simulink model "BiorlWalkingBipedRobot copy"  (R2023b)
settings: Solver=ode23t  StartTime=0.0  StopTime=inf  RelTol=1e-2  EnableMultiTasking=on
undefined symbols (not defined in the file or in its folder): foot_z, height_plane, init_angs_R, init_height, joint_stiffness, lower_leg_length, max_torque, plane_x, plane_y, Tf, Ts, upper_leg_length, wx0, wy0, X, Y, Z
libraries: sm_lib x38, nesl_utility x25, walkingRobotUtils x4, simulink x2, rllib x1
(part 1 of 2)
settings Model: Creator=The MathWorks, Inc.  LastModifiedBy=amelianelson
settings SolverCC: ZeroCrossAlgorithm=Adaptive  AlgebraicLoopSolver=TrustRegion
settings DataIOCC: SaveOutput=off  SignalLogging=off  DSMLogging=off  SaveTime=off  OutputTimes=0:0.01:10
settings OptimizationCC: LifeSpan=inf
settings DebuggingCC: MaxConsecutiveZCsMsg=warning  IgnoredZcDiagnostic=none  UnconnectedInputMsg=warning  UnconnectedOutputMsg=warning  UnconnectedLineMsg=warning  AllowSymbolicDim=off  SFUnexpectedBacktrackingDiag=warning  SFNoUnconditionalDefaultTransitionDiag=warning  SFExecutionAtInitializationDiag=none  UnitsInconsistencyMsg=none  ArithmeticOperatorsInVariantConditions=warning
settings ModelReferenceCC: EnableRefExpFcnMdlSchedulingChecks=on
settings SFSimCC: SimUseLocalCustomCode=off  CustomCodeUndefinedFunction=UseInterfaceOnly
settings RTWCC: RTWUseLocalCustomCode=off
settings CodeAppCC: StateflowObjectComments=on
settings GRTTargetCC: TargetLangStandard=C89/C90 (ANSI)
settings ConfigComp: CovMetricSettings=dw  CovSaveCumulativeToWorkspaceVar=on  CovSaveSingleToWorkspaceVar=on  CovExternalEMLEnable=off  CovSFcnEnable=off
settings SimscapeCC: SimscapeNormalizeSystem=off  SimscapeLogOpenViewer=on  SimscapeLogLimitData=off  SimscapeLogDataHistory=10000
settings ConfigurationSet: Description=SimMechanics 2G
settings DiagnosticsConfigSet: SimMechanicsRigidlyBoundBlock=none
settings ExplorerConfigSet: InternalSimMechanicsExplorerSettings="<ExplorerConfiguration><canonicalview>default</canonicalview><AnimationSetting><BasePlaybackSpeed>1.0</BasePlaybackSpeed><PlaybackSpeedFactor>1.0</PlaybackSpeedFactor></AnimationSetting><TilePanel><TileInfo><Tiles Columns=\"1\" Count=\"1\" Rows=\"1\"><Column Weight=\"1\"/><Row Weight=\"1\"/><Tile Height=\"1\" Width=\"1\" X=\"0\" Y=\"0\"/></Tiles></TileInfo><SceneInfo><SceneViewer><BGColor><R>0.60000002384185791</R><G>0.60000002384185791</G><B>0.60000002384185791</B></BGColor><Camera><DoPerspective>off</DoPerspective><Position><X>7.18002534815406079</X><Y>-8.21011991112170847</Y><Z>8.33180938462712462</Z></Position><Center><X>1.10741005252516134</X><Y>-0.176829942633513204</Y><Z>0.646464709811595872</Z></Center><Up><X>-0.335329266167064488</X><Y>0.506481739462631531</Y><Z>0.79437430147428989</Z></Up><ViewLimDist>1</ViewLimDist><YLim>0.739205014828661411</YLim><XLim>1.12849377732657596</XLim></Camera></SceneViewer></SceneInfo></TilePanel><MechEditorPanel><Cameras/><GfxPanelCameraMap/><VideoCreator><PlaybackSpeedRatio>1.0</PlaybackSpeedRatio><FrameRate>30</FrameRate><VideoFormat>Motion JPEG AVI</VideoFormat><FrameSize>auto</FrameSize></VideoCreator></MechEditorPanel></ExplorerConfiguration>"

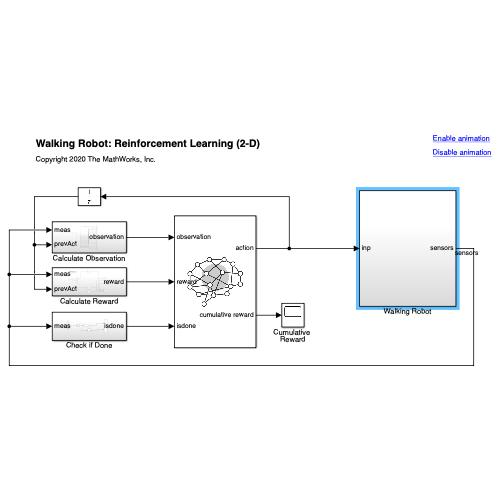
[thumbnail: Simulink's stored preview of the top-level diagram]
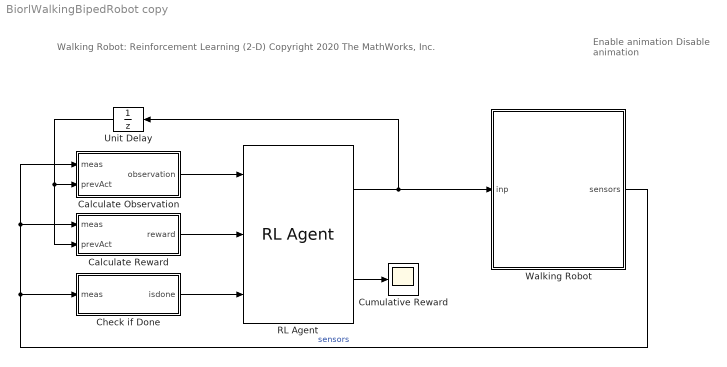
== system BiorlWalkingBipedRobot copy ==
  note: Enable animation
      |
      | Disable animation
  note: Walking Robot: Reinforcement Learning (2-D)
      |
      | Copyright 2020 The MathWorks, Inc.
  Calculate Observation : Subsystem
  Calculate Reward : Subsystem
  Check if Done : Subsystem
  Cumulative Reward : Scope
  RL Agent : rllib/RL Agent  Agent=agent  ExternalActionAsInput=off  ProvideLastAction=off  ProvideCumRwd=on  TreatAsDirectFeedthrough=on  UseStrictObservationDataTypes=off
  Unit Delay : UnitDelay  SampleTime=-1  HasFrameUpgradeWarning=on
  Walking Robot : Subsystem
  wires:
  Walking Robot/1(sensors) -> Calculate Reward/1(meas), Calculate Observation/1(meas), Check if Done/1(meas)  "sensors"
  Calculate Reward/1(reward) -> RL Agent/2
  Calculate Observation/1(observation) -> RL Agent/1
  Check if Done/1(isdone) -> RL Agent/3
  RL Agent/2 -> Cumulative Reward/1
  Unit Delay/1 -> Calculate Reward/2(prevAct), Calculate Observation/2(prevAct)
  RL Agent/1 -> Walking Robot/1(inp), Unit Delay/1

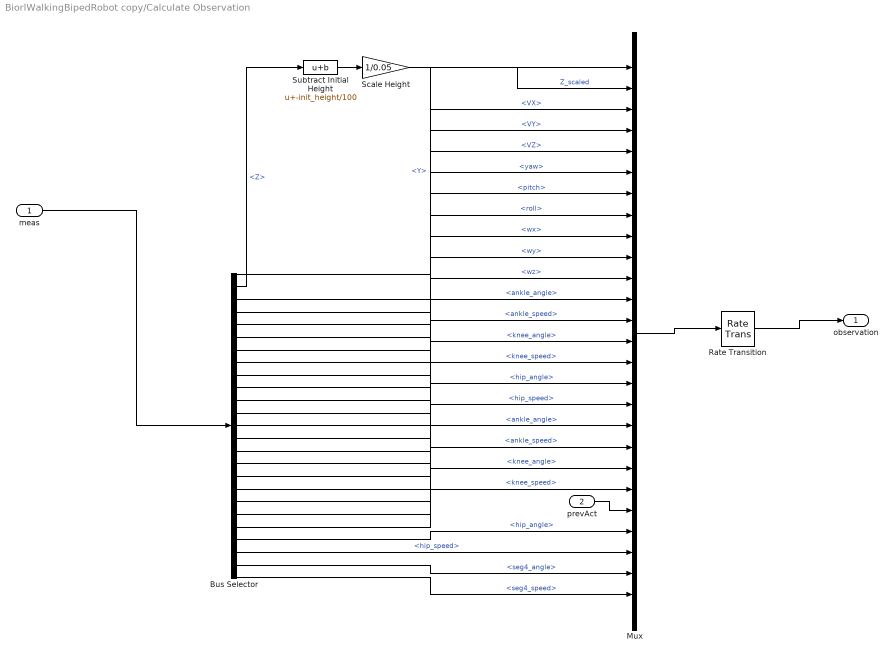
== system BiorlWalkingBipedRobot copy/Calculate Observation ==
  meas : Inport
  prevAct : Inport  Port=2
  Bus Selector : BusSelector  OutputSignals=Y,Z,VX,VY,VZ,yaw,pitch,roll,wx,wy,wz,measR.ankle_angle,measR.ankle_speed,measR.knee_angle,measR.knee_speed,measR.hip_angle,measR.hip_speed,measR.ankle_angle,measR.ankle_speed,measR.knee_angle,measR.knee_speed,measR.hip_angle,measR.hip_speed,measR.seg4_angle,measR.seg4_speed
  Mux : Mux  Inputs=26
  Rate Transition : RateTransition
  Scale Height : Gain  Gain=1/0.05
  Subtract Initial Height : Bias  Bias=-init_height/100  SaturateOnIntegerOverflow=off
  observation : Outport  VectorParamsAs1DForOutWhenUnconnected=off
  wires:
  meas/1 -> Bus Selector/1
  Mux/1 -> Rate Transition/1
  Rate Transition/1 -> observation/1
  prevAct/1 -> Mux/22
  Bus Selector/2 -> Subtract Initial Height/1  "<Z>"
  Subtract Initial Height/1 -> Scale Height/1
  Scale Height/1 -> Mux/2  "Z_scaled"
  Bus Selector/1 -> Mux/1  "<Y>"
  Bus Selector/4 -> Mux/4  "<VY>"
  Bus Selector/5 -> Mux/5  "<VZ>"
  Bus Selector/3 -> Mux/3  "<VX>"
  Bus Selector/6 -> Mux/6  "<yaw>"
  Bus Selector/7 -> Mux/7  "<pitch>"
  Bus Selector/8 -> Mux/8  "<roll>"
  Bus Selector/9 -> Mux/9  "<wx>"
  Bus Selector/10 -> Mux/10  "<wy>"
  Bus Selector/11 -> Mux/11  "<wz>"
  Bus Selector/12 -> Mux/12  "<ankle_angle>"
  Bus Selector/13 -> Mux/13  "<ankle_speed>"
  Bus Selector/14 -> Mux/14  "<knee_angle>"
  Bus Selector/15 -> Mux/15  "<knee_speed>"
  Bus Selector/16 -> Mux/16  "<hip_angle>"
  Bus Selector/17 -> Mux/17  "<hip_speed>"
  Bus Selector/18 -> Mux/18  "<ankle_angle>"
  Bus Selector/19 -> Mux/19  "<ankle_speed>"
  Bus Selector/20 -> Mux/20  "<knee_angle>"
  Bus Selector/21 -> Mux/21  "<knee_speed>"
  Bus Selector/22 -> Mux/23  "<hip_angle>"
  Bus Selector/23 -> Mux/24  "<hip_speed>"
  Bus Selector/24 -> Mux/25  "<seg4_angle>"
  Bus Selector/25 -> Mux/26  "<seg4_speed>"

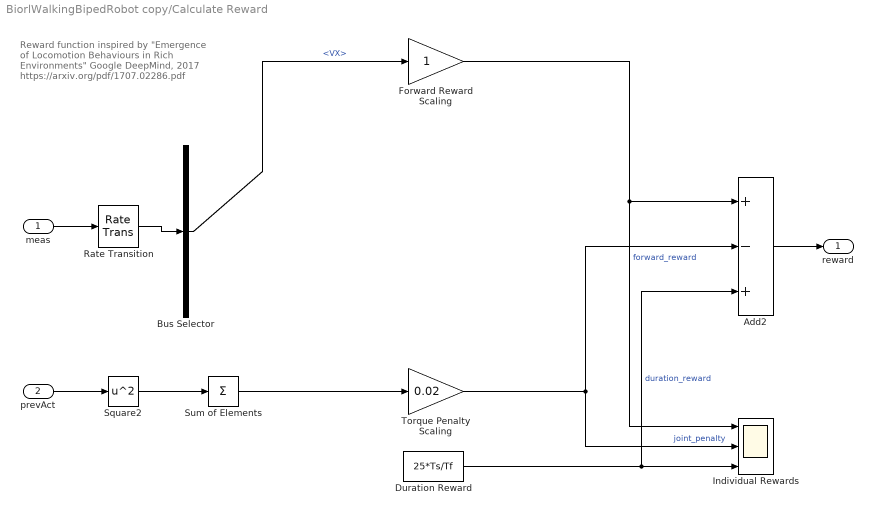
== system BiorlWalkingBipedRobot copy/Calculate Reward ==
  note: Reward function inspired by
      | "Emergence of Locomotion Behaviours in Rich Environments"
      | Google DeepMind, 2017
      | https://arxiv.org/pdf/1707.02286.pdf
  meas : Inport
  prevAct : Inport  Port=2
  Add2 : Sum  Inputs=+-+
  Bus Selector : BusSelector  OutputSignals=VX
  Duration Reward : Constant  Value=25*Ts/Tf
  Forward Reward Scaling : Gain
  Individual Rewards : Scope  NumInputPorts=3
  Rate Transition : RateTransition  OutPortSampleTime=Ts
  Square2 : Math  Operator=square  SignedPower=on
  Sum of Elements : Sum  Inputs=+
  Torque Penalty Scaling : Gain  Gain=0.02
  reward : Outport  VectorParamsAs1DForOutWhenUnconnected=off
  wires:
  meas/1 -> Rate Transition/1
  Rate Transition/1 -> Bus Selector/1
  Add2/1 -> reward/1
  Forward Reward Scaling/1 -> Add2/1, Individual Rewards/1  "forward_reward"
  Sum of Elements/1 -> Torque Penalty Scaling/1
  Bus Selector/1 -> Forward Reward Scaling/1  "<VX>"
  Duration Reward/1 -> Individual Rewards/3, Add2/3  "duration_reward"
  prevAct/1 -> Square2/1
  Square2/1 -> Sum of Elements/1
  Torque Penalty Scaling/1 -> Add2/2, Individual Rewards/2  "joint_penalty"

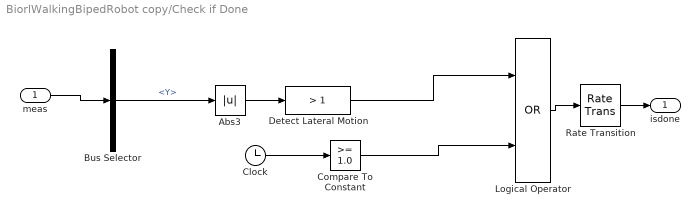
== system BiorlWalkingBipedRobot copy/Check if Done ==
  meas : Inport
  Abs3 : Abs  SaturateOnIntegerOverflow=off
  Bus Selector : BusSelector  OutputSignals=Y
  Clock : Clock
  Compare To Constant : simulink/Logic and Bit Operations/Compare To Constant  relop=>=  const=1.0  OutDataTypeStr=boolean
  Detect Lateral Motion : simulink/Logic and Bit Operations/Compare To Constant  relop=>  const=1  OutDataTypeStr=boolean
  Logical Operator : Logic  Operator=OR  AllPortsSameDT=off  OutDataTypeStr=boolean
  Rate Transition : RateTransition
  isdone : Outport  VectorParamsAs1DForOutWhenUnconnected=off
  wires:
  Logical Operator/1 -> Rate Transition/1
  meas/1 -> Bus Selector/1
  Rate Transition/1 -> isdone/1
  Bus Selector/1 -> Abs3/1  "<Y>"
  Detect Lateral Motion/1 -> Logical Operator/1
  Abs3/1 -> Detect Lateral Motion/1
  Clock/1 -> Compare To Constant/1
  Compare To Constant/1 -> Logical Operator/2

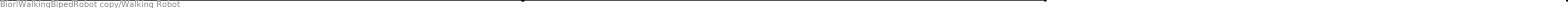
== system BiorlWalkingBipedRobot copy/Walking Robot ==
  note: masks_array
  note: 3 torques per leg
      | (ankle knee hip)
  inp : Inport
  6-DOF Joint : sm_lib/Joints/6-DOF Joint  JointMode=Normal  SenseConstraintForce=off  SenseConstraintForceX=off  SenseConstraintForceY=off  SenseConstraintForceZ=off  SenseConstraintTorque=off  SenseConstraintTorqueX=off  SenseConstraintTorqueY=off  SenseConstraintTorqueZ=off  SenseTotalForce=off  SenseTotalForceX=off  SenseTotalForceY=off  SenseTotalForceZ=off  SenseTotalTorque=off  SenseTotalTorqueX=off  SenseTotalTorqueY=off  SenseTotalTorqueZ=off  CompositeWrenchDir=FollowerOnBase  CompositeWrenchFrame=BaseFrame  PxEquilibriumPosition=0  PxEquilibriumPositionUnits=m  PxSpringStiffness=0  PxSpringStiffnessUnits=N/m  PxDampingCoefficient=world_damping  PxDampingCoefficientUnits=N/(m/s)  PxTorqueActuationMode=NoTorque  PxMotionActuationMode=ComputedMotion  PxSensePosition=off  PxSenseVelocity=off  PxSenseAcceleration=off  PxSenseTorqueForce=off  PxSenseLowerLimitTorqueForce=off  PxSenseUpperLimitTorqueForce=off  PxLowerLimitSpecify=off  PxLowerLimitBound=-1  PxLowerLimitBoundUnits=m  PxLowerLimitStiffness=1e6  PxLowerLimitStiffnessUnits=N/m  PxLowerLimitDamping=1e3  PxLowerLimitDampingUnits=N/(m/s)  PxLowerLimitTransitionRegionWidth=1e-4  PxLowerLimitTransitionRegionWidthUnits=m  PxUpperLimitSpecify=off  PxUpperLimitBound=1  PxUpperLimitBoundUnits=m  PxUpperLimitStiffness=1e6  PxUpperLimitStiffnessUnits=N/m  PxUpperLimitDamping=1e3  PxUpperLimitDampingUnits=N/(m/s)  PxUpperLimitTransitionRegionWidth=1e-4  PxUpperLimitTransitionRegionWidthUnits=m  PxPositionTargetSpecify=on  PxPositionTargetPriority=High  PxPositionTargetValue=0  PxPositionTargetValueUnits=m  PxVelocityTargetSpecify=on  PxVelocityTargetPriority=High  PxVelocityTargetValue=vx0  PxVelocityTargetValueUnits=m/s  PyEquilibriumPosition=0  PyEquilibriumPositionUnits=m  PySpringStiffness=0  PySpringStiffnessUnits=N/m  PyDampingCoefficient=world_damping  PyDampingCoefficientUnits=N/(m/s)  PyTorqueActuationMode=NoTorque  PyMotionActuationMode=ComputedMotion  PySensePosition=off  PySenseVelocity=off  PySenseAcceleration=off  PySenseTorqueForce=off  PySenseLowerLimitTorqueForce=off  PySenseUpperLimitTorqueForce=off  PyLowerLimitSpecify=off  PyLowerLimitBound=-1  PyLowerLimitBoundUnits=m  PyLowerLimitStiffness=1e6  PyLowerLimitStiffnessUnits=N/m  PyLowerLimitDamping=1e3  PyLowerLimitDampingUnits=N/(m/s)  PyLowerLimitTransitionRegionWidth=1e-4  PyLowerLimitTransitionRegionWidthUnits=m  PyUpperLimitSpecify=off  PyUpperLimitBound=1  PyUpperLimitBoundUnits=m  PyUpperLimitStiffness=1e6  PyUpperLimitStiffnessUnits=N/m  PyUpperLimitDamping=1e3  PyUpperLimitDampingUnits=N/(m/s)  PyUpperLimitTransitionRegionWidth=1e-4  PyUpperLimitTransitionRegionWidthUnits=m  PyPositionTargetSpecify=on  PyPositionTargetPriority=High  PyPositionTargetValue=0  PyPositionTargetValueUnits=m  PyVelocityTargetSpecify=on  PyVelocityTargetPriority=High  PyVelocityTargetValue=0  PyVelocityTargetValueUnits=m/s  PzEquilibriumPosition=0  PzEquilibriumPositionUnits=m  PzSpringStiffness=0  PzSpringStiffnessUnits=N/m  PzDampingCoefficient=world_damping  PzDampingCoefficientUnits=N/(m/s)  PzTorqueActuationMode=NoTorque  PzMotionActuationMode=ComputedMotion  PzSensePosition=off  PzSenseVelocity=off  PzSenseAcceleration=off  PzSenseTorqueForce=off  PzSenseLowerLimitTorqueForce=off  PzSenseUpperLimitTorqueForce=off  PzLowerLimitSpecify=off  PzLowerLimitBound=-1  PzLowerLimitBoundUnits=m  PzLowerLimitStiffness=1e6  PzLowerLimitStiffnessUnits=N/m  PzLowerLimitDamping=1e3  PzLowerLimitDampingUnits=N/(m/s)  PzLowerLimitTransitionRegionWidth=1e-4  PzLowerLimitTransitionRegionWidthUnits=m  PzUpperLimitSpecify=off  PzUpperLimitBound=1  PzUpperLimitBoundUnits=m  PzUpperLimitStiffness=1e6  PzUpperLimitStiffnessUnits=N/m  PzUpperLimitDamping=1e3  PzUpperLimitDampingUnits=N/(m/s)  PzUpperLimitTransitionRegionWidth=1e-4  PzUpperLimitTransitionRegionWidthUnits=m  PzPositionTargetSpecify=on  PzPositionTargetPriority=High  PzPositionTargetValue=init_height  PzPositionTargetValueUnits=cm  PzVelocityTargetSpecify=off  PzVelocityTargetPriority=High  PzVelocityTargetValue=0  PzVelocityTargetValueUnits=m/s  SphEqPosRotationMethod=None  SphEqPosRotationAngleUnits=deg  SphEqPosRotationStandardAxis=+Z  SphEqPosRotationAngle=0.0  SphEqPosRotationArbitraryAxis=[0 0 1]  SphEqPosFollAlignAxisA=+X  SphEqPosBaseAlignAxisA=+Y  SphEqPosFollAlignAxisB=+Y  SphEqPosBaseAlignAxisB=+Z  SphEqPosRotationSequenceAxes=FollowerAxes  SphEqPosRotationSequence=XYX  SphEqPosRotationSequenceAngles=[0 0 0]  SphEqPosRotationSequenceAnglesUnits=deg  SphEqPosRotationMatrix=[1 0 0; 0 1 0; 0 0 1]  SphEqPosQuaternion=[1 0 0 0]  SphSpringStiffness=0  SphSpringStiffnessUnits=N*m/deg  SphDampingCoefficient=world_rot_damping  SphDampingCoefficientUnits=N*m/(rad/s)  SphActuateTorqueX=off  SphActuateTorqueY=off  SphActuateTorqueZ=off  SphActuateTorque=off  SphTorqueActuationMode=NoTorque  SphMotionActuationMode=ComputedMotion  SphActuationFrame=BaseFrame  SphSensePosition=off  SphSenseVelocityX=off  SphSenseVelocityY=off  SphSenseVelocityZ=off  SphSenseVelocity=off  SphSenseAccelerationX=off  SphSenseAccelerationY=off  SphSenseAccelerationZ=off  SphSenseAcceleration=off  SphSenseTorqueX=off  SphSenseTorqueY=off  SphSenseTorqueZ=off  SphSenseTorqueForce=off  SphSenseLowerLimitTorqueMag=off  SphSenseUpperLimitTorqueMag=off  SphSensingFrame=BaseFrame  SphLowerLimitSpecify=off  SphLowerLimitBound=15  SphLowerLimitBoundUnits=deg  SphLowerLimitStiffness=1e4  SphLowerLimitStiffnessUnits=N*m/deg  SphLowerLimitDamping=10  SphLowerLimitDampingUnits=N*m/(deg/s)  SphLowerLimitTransitionRegionWidth=0.1  SphLowerLimitTransitionRegionWidthUnits=deg  SphUpperLimitSpecify=off  SphUpperLimitBound=45  SphUpperLimitBoundUnits=deg  SphUpperLimitStiffness=1e4  SphUpperLimitStiffnessUnits=N*m/deg  SphUpperLimitDamping=10  SphUpperLimitDampingUnits=N*m/(deg/s)  SphUpperLimitTransitionRegionWidth=0.1  SphUpperLimitTransitionRegionWidthUnits=deg  SphPositionTargetRotationMethod=RotationSequence  SphPositionTargetRotationAngleUnits=deg  SphPositionTargetRotationStandardAxis=+Z  SphPositionTargetRotationAngle=0.0  SphPositionTargetRotationArbitraryAxis=[0 0 1]  SphPositionTargetFollAlignAxisA=+X  SphPositionTargetBaseAlignAxisA=+Y  SphPositionTargetFollAlignAxisB=+Y  SphPositionTargetBaseAlignAxisB=+Z  SphPositionTargetRotationSequenceAxes=FollowerAxes  SphPositionTargetRotationSequence=XYX  SphPositionTargetRotationSequenceAngles=[wx0 wy0 0]  SphPositionTargetRotationSequenceAnglesUnits=rad  SphPositionTargetRotationMatrix=eye(3)  SphPositionTargetQuaternion=[1 0 0 0]  SphPositionTargetSpecify=on  SphPositionTargetPriority=High  SphVelocityTargetValue=[0 0 0]  SphVelocityTargetValueUnits=deg/s  SphVelocityTargetSpecify=off  SphVelocityTargetPriority=High  SphVelocityTargetInFollowerFrame=on
  Actions : Scope
  Demux : Demux  Outputs=1
  Right Hip to Torso : sm_lib/Frames and Transforms/Rigid Transform  TranslationMethod=Cartesian  TranslationStandardOffset=0  TranslationStandardOffsetUnits=cm  TranslationStandardAxis=+Z  TranslationCartesianOffset=[0 0 0]  TranslationCartesianOffsetUnits=cm  TranslationROffset=0  TranslationROffsetUnits=m  TranslationZOffset=0  TranslationZOffsetUnits=m  TranslationThetaOffset=0  TranslationThetaOffsetUnits=deg  RotationMethod=None  RotationAngleUnits=deg  RotationStandardAxis=+Z  RotationAngle=0.0  RotationArbitraryAxis=[0 0 1]  FollAlignAxisA=+X  BaseAlignAxisA=+Y  FollAlignAxisB=+Y  BaseAlignAxisB=+Z  RotationSequenceAxes=FollowerAxes  RotationSequence=XYX  RotationSequenceAngles=[0 0 0]  RotationSequenceAnglesUnits=deg  RotationMatrix=[1 0 0; 0 1 0; 0 0 1]  Quaternion=[1 0 0 0]
  Robot Leg R : Subsystem
  Sensors : Subsystem
  Spatial Contact Force : sm_lib/Forces and Torques/Spatial Contact Force  SenseContactBaseRotation=off  SenseContactBaseTranslation=off  CoefficientOfDynamicFriction=mu_k  CoefficientOfStaticFriction=mu_s  NormalDamping=contact_damping  NormalDampingUnits=N/(m/s)  SenseContactSignal=off  NormalStiffness=contact_stiffness  NormalStiffnessUnits=N/m  FrictionalCriticalVelocity=mu_vth  FrictionalCriticalVelocityUnits=m/s  ZeroCrossDetectContactStartAndEnd=off  SenseContactFollowerRotation=off  SenseContactFollowerTranslation=off  FrictionType=SmoothStickSlip  SenseFrictionalForceMagnitude=on  SenseNormalForceMagnitude=on  NormalForceType=SmoothSpringDamper  SenseNormalVelocity=off  SensePenetrationDepth=off  SenseSeparationDistance=off  SenseTangentialVelocity=off  NormalTransitionRegionWidth=1e-4  NormalTransitionRegionWidthUnits=m
  Spherical Solid : sm_lib/Body Elements/Spherical Solid  GraphicAmbientColor=[0.15 0.15 0.15 1.0]  BasedOnType=Mass  CenterOfMass=[0 0 0]  CenterOfMassUnits=m  GraphicDiffuseColor=[0.5 0.5 0.5]  Density=1000  DensityUnits=kg/m^3  DoExposeReferenceFrame=on  GraphicEmissiveColor=[0.0 0.0 0.0 1.0]  ExportEntireGeometry=on  SerializedExposedGeometries=<ExposedGeometries><ExposedGeometry><RawGeometryId>entire</RawGeometryId><ExposedGeometryId>G</ExposedGeometryId></ExposedGeometry></ExposedGeometries>  SerializedFrames=<Frames/>  MarkerShape=Sphere  MarkerSize=10  GraphicType=FromGeometry  InertiaType=CalculateFromGeometry  Mass=1  MassUnits=g  MomentsOfInertia=[1 1 1]  MomentsOfInertiaUnits=kg*m^2  GraphicOpacity=1.0  ProductsOfInertia=[0 0 0]  ProductsOfInertiaUnits=kg*m^2  GraphicShininess=75  GraphicSpecularColor=[0.5 0.5 0.5 1.0]  SphereRadius=foot_z/2  SphereRadiusUnits=cm  GraphicVisPropType=SimpleVisualProperties
  Spline : sm_lib/Curves and Surfaces/Spline  GraphicAmbientColor=[0.15 0.15 0.15 1.0]  GraphicDiffuseColor=[0 0 0]  DataPoints=[0 0 0.025; 5 0 0.025]  DataPointsUnits=m  GraphicEmissiveColor=[0.0 0.0 0.0 1.0]  EndConditionType=Natural  MarkerShape=Sphere  MarkerSize=10  GraphicType=FromGeometry  GraphicOpacity=1.0  GraphicShininess=75  GraphicSpecularColor=[0.5 0.5 0.5 1.0]  GraphicVisPropType=SimpleVisualProperties
  Torque Scaling : Gain  Gain=max_torque
  Torso : sm_lib/Body Elements/Brick Solid  GraphicAmbientColor=[0.15 0.15 0.15 1.0]  BasedOnType=Density  BrickDimensions=[1 1 1]  BrickDimensionsUnits=cm  CenterOfMass=[0 0 0]  CenterOfMassUnits=m  GraphicDiffuseColor=[0.5 0.5 0.5]  Density=density  DensityUnits=kg/m^3  DoExposeReferenceFrame=on  GraphicEmissiveColor=[0.0 0.0 0.0 1.0]  ExportEntireGeometry=off  SerializedFrames=<Frames><Frame><Id>Frame1</Id><Value><Name>F1</Name><Origin><Source>CenterOfMassFrame</Source><FeatureName></FeatureName></Origin><PrimaryAxis><DefinedDirection>+Z</DefinedDirection><Source>ReferenceFrame</Source><SourceDirection>+Z</SourceDirection><FeatureName></FeatureName></PrimaryAxis><SecondaryAxis><DefinedDirection>+X</DefinedDirection><Source>ReferenceFrame</Source><SourceDirection>+X</SourceDirection><FeatureName></FeatureName></SecondaryAxis></Value></Frame></Frames>  MarkerShape=Sphere  MarkerSize=10  GraphicType=FromGeometry  InertiaType=CalculateFromGeometry  Mass=1  MassUnits=kg  MomentsOfInertia=[1 1 1]  MomentsOfInertiaUnits=kg*m^2  GraphicOpacity=1.0  ProductsOfInertia=[1 1 1]  ProductsOfInertiaUnits=kg*m^2  GraphicShininess=75  GraphicSpecularColor=[0.5 0.5 0.5 1.0]  GraphicVisPropType=SimpleVisualProperties
  World and Ground : Subsystem
  sensors : Outport  VectorParamsAs1DForOutWhenUnconnected=off
  wires:
  Robot Leg R/1(meas) -> Sensors/1(measR)
  Sensors/1(sensors) -> sensors/1
  Demux/1 -> Robot Leg R/1(torques), Actions/1  "right_torques"
  Torque Scaling/1 -> Demux/1
  inp/1 -> Torque Scaling/1
  connections:
  Spline/LConn1 -- Sensors/LConn1 -- 6-DOF Joint/LConn1 -- World and Ground/LConn1
  Robot Leg R/RConn2 -- Spatial Contact Force/LConn1 -- World and Ground/RConn1
  Robot Leg R/RConn1 -- Right Hip to Torso/RConn1
  6-DOF Joint/RConn1 -- Torso/RConn1 -- Sensors/RConn1 -- Right Hip to Torso/LConn1
  ?
  ?
  ?
  ?
  ?
  ?
  ?
  Spherical Solid/LConn1 -- Spatial Contact Force/RConn1
  Spherical Solid/RConn1 -- Torso/LConn1

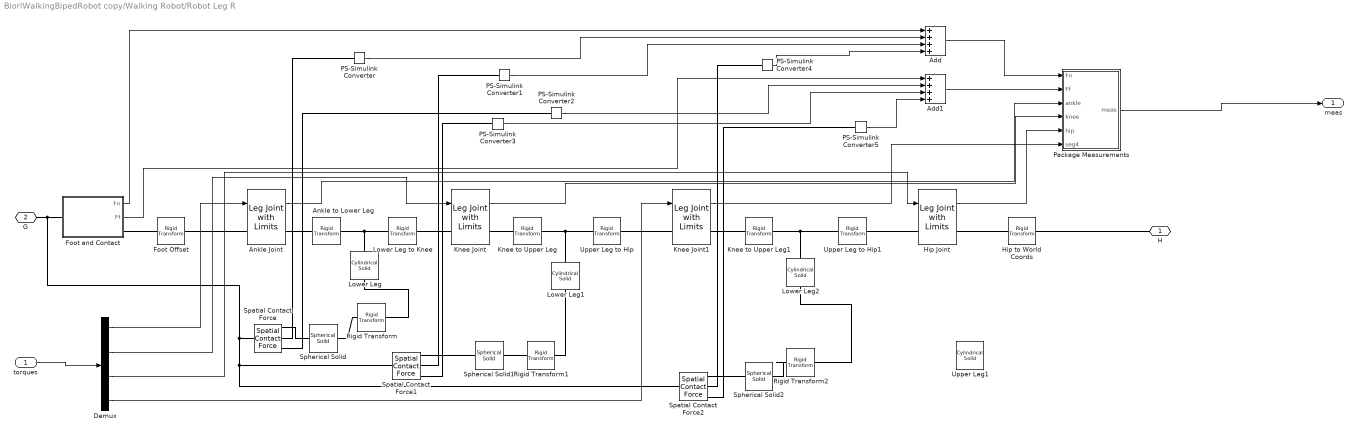
== system BiorlWalkingBipedRobot copy/Walking Robot/Robot Leg R ==
  torques : Inport
  Add : Sum  Inputs=++++
  Add1 : Sum  Inputs=++++
  Ankle Joint : walkingRobotUtils/Leg Joint with Limits  VariantControl=actuatorType == 2  k=joint_stiffness  d=joint_damping  initAngle=0  eqAngle=0  upperLimit=pi  lowerLimit=-pi  jointLimitStiffness=joint_limit_stiffness  jointLimitDamping=joint_limit_damping
  Ankle to Lower Leg : sm_lib/Frames and Transforms/Rigid Transform  TranslationMethod=Cartesian  TranslationStandardOffset=0  TranslationStandardOffsetUnits=cm  TranslationStandardAxis=+Z  TranslationCartesianOffset=[0 lower_leg_length/2 0]  TranslationCartesianOffsetUnits=cm  TranslationROffset=0  TranslationROffsetUnits=m  TranslationZOffset=0  TranslationZOffsetUnits=m  TranslationThetaOffset=0  TranslationThetaOffsetUnits=deg  RotationMethod=StandardAxis  RotationAngleUnits=deg  RotationStandardAxis=+X  RotationAngle=-90  RotationArbitraryAxis=[0 0 1]  FollAlignAxisA=+X  BaseAlignAxisA=+Y  FollAlignAxisB=+Y  BaseAlignAxisB=+Z  RotationSequenceAxes=FollowerAxes  RotationSequence=XYX  RotationSequenceAngles=[0 0 0]  RotationSequenceAnglesUnits=deg  RotationMatrix=[1 0 0; 0 1 0; 0 0 1]  Quaternion=[1 0 0 0]
  Demux : Demux
  Foot Offset : sm_lib/Frames and Transforms/Rigid Transform  TranslationMethod=Cartesian  TranslationStandardOffset=0  TranslationStandardOffsetUnits=cm  TranslationStandardAxis=+Z  TranslationCartesianOffset=[0 0 0]  TranslationCartesianOffsetUnits=cm  TranslationROffset=0  TranslationROffsetUnits=m  TranslationZOffset=0  TranslationZOffsetUnits=m  TranslationThetaOffset=0  TranslationThetaOffsetUnits=deg  RotationMethod=None  RotationAngleUnits=deg  RotationStandardAxis=+X  RotationAngle=-90  RotationArbitraryAxis=[0 0 1]  FollAlignAxisA=+X  BaseAlignAxisA=+Y  FollAlignAxisB=+Y  BaseAlignAxisB=+Z  RotationSequenceAxes=FollowerAxes  RotationSequence=XYX  RotationSequenceAngles=[0 0 0]  RotationSequenceAnglesUnits=deg  RotationMatrix=[1 0 0; 0 1 0; 0 0 1]  Quaternion=[1 0 0 0]
  Foot and Contact : Subsystem  AncestorBlock=walkingRobotUtils/Foot and Contact
  Hip Joint : walkingRobotUtils/Leg Joint with Limits  VariantControl=actuatorType == 2  k=joint_stiffness  d=joint_damping  initAngle=-init_angs_R(1)  eqAngle=0  upperLimit=pi/2  lowerLimit=-pi/2  jointLimitStiffness=joint_limit_stiffness  jointLimitDamping=joint_limit_damping
  Hip to World Coords : sm_lib/Frames and Transforms/Rigid Transform  TranslationMethod=None  TranslationStandardOffset=0  TranslationStandardOffsetUnits=cm  TranslationStandardAxis=+Z  TranslationCartesianOffset=[0 0 upper_leg_length/2]  TranslationCartesianOffsetUnits=cm  TranslationROffset=0  TranslationROffsetUnits=m  TranslationZOffset=0  TranslationZOffsetUnits=m  TranslationThetaOffset=0  TranslationThetaOffsetUnits=deg  RotationMethod=StandardAxis  RotationAngleUnits=deg  RotationStandardAxis=+X  RotationAngle=-90  RotationArbitraryAxis=[0 0 1]  FollAlignAxisA=+X  BaseAlignAxisA=+Y  FollAlignAxisB=+Y  BaseAlignAxisB=+Z  RotationSequenceAxes=FollowerAxes  RotationSequence=XYX  RotationSequenceAngles=[0 0 0]  RotationSequenceAnglesUnits=deg  RotationMatrix=[1 0 0; 0 1 0; 0 0 1]  Quaternion=[1 0 0 0]
  Knee Joint : walkingRobotUtils/Leg Joint with Limits  VariantControl=actuatorType == 2  k=joint_stiffness  d=joint_damping  initAngle=init_angs_R(2)  eqAngle=0  upperLimit=pi/2  lowerLimit=-pi/2  jointLimitStiffness=joint_limit_stiffness  jointLimitDamping=joint_limit_damping
  Knee Joint1 : walkingRobotUtils/Leg Joint with Limits  VariantControl=actuatorType == 2  k=joint_stiffness  d=joint_damping  initAngle=init_angs_R(2)  eqAngle=0  upperLimit=pi/2  lowerLimit=-pi/2  jointLimitStiffness=joint_limit_stiffness  jointLimitDamping=joint_limit_damping
  Knee to Upper Leg : sm_lib/Frames and Transforms/Rigid Transform  TranslationMethod=Cartesian  TranslationStandardOffset=0  TranslationStandardOffsetUnits=cm  TranslationStandardAxis=+Z  TranslationCartesianOffset=[0 upper_leg_length/2 0]  TranslationCartesianOffsetUnits=cm  TranslationROffset=0  TranslationROffsetUnits=m  TranslationZOffset=0  TranslationZOffsetUnits=m  TranslationThetaOffset=0  TranslationThetaOffsetUnits=deg  RotationMethod=StandardAxis  RotationAngleUnits=deg  RotationStandardAxis=+X  RotationAngle=-90  RotationArbitraryAxis=[0 0 1]  FollAlignAxisA=+X  BaseAlignAxisA=+Y  FollAlignAxisB=+Y  BaseAlignAxisB=+Z  RotationSequenceAxes=FollowerAxes  RotationSequence=XYX  RotationSequenceAngles=[0 0 0]  RotationSequenceAnglesUnits=deg  RotationMatrix=[1 0 0; 0 1 0; 0 0 1]  Quaternion=[1 0 0 0]
  Knee to Upper Leg1 : sm_lib/Frames and Transforms/Rigid Transform  TranslationMethod=Cartesian  TranslationStandardOffset=0  TranslationStandardOffsetUnits=cm  TranslationStandardAxis=+Z  TranslationCartesianOffset=[0 upper_leg_length/2 0]  TranslationCartesianOffsetUnits=cm  TranslationROffset=0  TranslationROffsetUnits=m  TranslationZOffset=0  TranslationZOffsetUnits=m  TranslationThetaOffset=0  TranslationThetaOffsetUnits=deg  RotationMethod=StandardAxis  RotationAngleUnits=deg  RotationStandardAxis=+X  RotationAngle=-90  RotationArbitraryAxis=[0 0 1]  FollAlignAxisA=+X  BaseAlignAxisA=+Y  FollAlignAxisB=+Y  BaseAlignAxisB=+Z  RotationSequenceAxes=FollowerAxes  RotationSequence=XYX  RotationSequenceAngles=[0 0 0]  RotationSequenceAnglesUnits=deg  RotationMatrix=[1 0 0; 0 1 0; 0 0 1]  Quaternion=[1 0 0 0]
  Lower Leg : sm_lib/Body Elements/Cylindrical Solid  GraphicAmbientColor=[0.15 0.15 0.15 1.0]  BasedOnType=Density  CenterOfMass=[0 0 0]  CenterOfMassUnits=m  GraphicDiffuseColor=[0.4 0.4 1.0]  CylinderLength=lower_leg_length  CylinderLengthUnits=cm  CylinderRadius=leg_radius  CylinderRadiusUnits=cm  Density=density  DensityUnits=kg/m^3  DoExposeReferenceFrame=on  GraphicEmissiveColor=[0.0 0.0 0.0 1.0]  ExportEntireGeometry=off  SerializedFrames=<Frames><Frame><Id>Frame1</Id><Value><Name>F1</Name><Origin><Source>GeometricFeature</Source><FeatureName>top surface</FeatureName></Origin><PrimaryAxis><DefinedDirection>+Z</DefinedDirection><Source>ReferenceFrame</Source><SourceDirection>+Z</SourceDirection><FeatureName></FeatureName></PrimaryAxis><SecondaryAxis><DefinedDirection>+X</DefinedDirection><Source>ReferenceFrame</Source><SourceDirection>+X</SourceDirection><FeatureName></FeatureName></SecondaryAxis></Value></Frame></Frames>  MarkerShape=Sphere  MarkerSize=10  GraphicType=FromGeometry  InertiaType=CalculateFromGeometry  Mass=1  MassUnits=kg  MomentsOfInertia=[1 1 1]  MomentsOfInertiaUnits=kg*m^2  GraphicOpacity=1.0  ProductsOfInertia=[1 1 1]  ProductsOfInertiaUnits=kg*m^2  GraphicShininess=75  GraphicSpecularColor=[0.5 0.5 0.5 1.0]  GraphicVisPropType=SimpleVisualProperties
  Lower Leg to Knee : sm_lib/Frames and Transforms/Rigid Transform  TranslationMethod=Cartesian  TranslationStandardOffset=0  TranslationStandardOffsetUnits=cm  TranslationStandardAxis=+Z  TranslationCartesianOffset=[0 0 lower_leg_length/2]  TranslationCartesianOffsetUnits=cm  TranslationROffset=0  TranslationROffsetUnits=m  TranslationZOffset=0  TranslationZOffsetUnits=m  TranslationThetaOffset=0  TranslationThetaOffsetUnits=deg  RotationMethod=StandardAxis  RotationAngleUnits=deg  RotationStandardAxis=+X  RotationAngle=90  RotationArbitraryAxis=[0 0 1]  FollAlignAxisA=+X  BaseAlignAxisA=+Y  FollAlignAxisB=+Y  BaseAlignAxisB=+Z  RotationSequenceAxes=FollowerAxes  RotationSequence=XYX  RotationSequenceAngles=[0 0 0]  RotationSequenceAnglesUnits=deg  RotationMatrix=[1 0 0; 0 1 0; 0 0 1]  Quaternion=[1 0 0 0]
  Lower Leg1 : sm_lib/Body Elements/Cylindrical Solid  GraphicAmbientColor=[0.15 0.15 0.15 1.0]  BasedOnType=Density  CenterOfMass=[0 0 0]  CenterOfMassUnits=m  GraphicDiffuseColor=[1.0 0.2 0.0]  CylinderLength=lower_leg_length  CylinderLengthUnits=cm  CylinderRadius=leg_radius  CylinderRadiusUnits=cm  Density=density  DensityUnits=kg/m^3  DoExposeReferenceFrame=on  GraphicEmissiveColor=[0.0 0.0 0.0 1.0]  ExportEntireGeometry=off  SerializedFrames=<Frames><Frame><Id>Frame1</Id><Value><Name>F1</Name><Origin><Source>GeometricFeature</Source><FeatureName>top surface</FeatureName></Origin><PrimaryAxis><DefinedDirection>+Z</DefinedDirection><Source>ReferenceFrame</Source><SourceDirection>+Z</SourceDirection><FeatureName></FeatureName></PrimaryAxis><SecondaryAxis><DefinedDirection>+X</DefinedDirection><Source>ReferenceFrame</Source><SourceDirection>+X</SourceDirection><FeatureName></FeatureName></SecondaryAxis></Value></Frame></Frames>  MarkerShape=Sphere  MarkerSize=10  GraphicType=FromGeometry  InertiaType=CalculateFromGeometry  Mass=1  MassUnits=kg  MomentsOfInertia=[1 1 1]  MomentsOfInertiaUnits=kg*m^2  GraphicOpacity=1.0  ProductsOfInertia=[1 1 1]  ProductsOfInertiaUnits=kg*m^2  GraphicShininess=75  GraphicSpecularColor=[0.5 0.5 0.5 1.0]  GraphicVisPropType=SimpleVisualProperties
  Lower Leg2 : sm_lib/Body Elements/Cylindrical Solid  GraphicAmbientColor=[0.15 0.15 0.15 1.0]  BasedOnType=Density  CenterOfMass=[0 0 0]  CenterOfMassUnits=m  GraphicDiffuseColor=[0.6 0.0 0.6]  CylinderLength=lower_leg_length  CylinderLengthUnits=cm  CylinderRadius=leg_radius  CylinderRadiusUnits=cm  Density=density  DensityUnits=kg/m^3  DoExposeReferenceFrame=on  GraphicEmissiveColor=[0.0 0.0 0.0 1.0]  ExportEntireGeometry=off  SerializedFrames=<Frames><Frame><Id>Frame1</Id><Value><Name>F1</Name><Origin><Source>GeometricFeature</Source><FeatureName>top surface</FeatureName></Origin><PrimaryAxis><DefinedDirection>+Z</DefinedDirection><Source>ReferenceFrame</Source><SourceDirection>+Z</SourceDirection><FeatureName></FeatureName></PrimaryAxis><SecondaryAxis><DefinedDirection>+X</DefinedDirection><Source>ReferenceFrame</Source><SourceDirection>+X</SourceDirection><FeatureName></FeatureName></SecondaryAxis></Value></Frame></Frames>  MarkerShape=Sphere  MarkerSize=10  GraphicType=FromGeometry  InertiaType=CalculateFromGeometry  Mass=1  MassUnits=kg  MomentsOfInertia=[1 1 1]  MomentsOfInertiaUnits=kg*m^2  GraphicOpacity=1.0  ProductsOfInertia=[1 1 1]  ProductsOfInertiaUnits=kg*m^2  GraphicShininess=75  GraphicSpecularColor=[0.5 0.5 0.5 1.0]  GraphicVisPropType=SimpleVisualProperties
  PS-Simulink Converter{,1..5} (6 alike) : nesl_utility/PS-Simulink Converter  PhysicalDomain=network_engine_domain  SubClassName=ps_output  LeftPortType=input  RightPortType=output  PseudoPeriodic=off  Frequencies=[]  VectorFormat=inherit  Unit=inherit  AffineConversion=off
  Package Measurements : Subsystem  AncestorBlock="walkingRobotUtils/Package  Measurements 2D"
  Rigid Transform : sm_lib/Frames and Transforms/Rigid Transform  TranslationMethod=None  TranslationStandardOffset=0  TranslationStandardOffsetUnits=m  TranslationStandardAxis=+Z  TranslationCartesianOffset=[0 0 0]  TranslationCartesianOffsetUnits=m  TranslationROffset=0  TranslationROffsetUnits=m  TranslationZOffset=0  TranslationZOffsetUnits=m  TranslationThetaOffset=0  TranslationThetaOffsetUnits=deg  RotationMethod=None  RotationAngleUnits=deg  RotationStandardAxis=+Z  RotationAngle=0.0  RotationArbitraryAxis=[0 0 1]  FollAlignAxisA=+X  BaseAlignAxisA=+Y  FollAlignAxisB=+Y  BaseAlignAxisB=+Z  RotationSequenceAxes=FollowerAxes  RotationSequence=XYX  RotationSequenceAngles=[0 0 0]  RotationSequenceAnglesUnits=deg  RotationMatrix=[1 0 0; 0 1 0; 0 0 1]  Quaternion=[1 0 0 0]
  Rigid Transform1 : sm_lib/Frames and Transforms/Rigid Transform  TranslationMethod=None  TranslationStandardOffset=0  TranslationStandardOffsetUnits=m  TranslationStandardAxis=+Z  TranslationCartesianOffset=[0 0 0]  TranslationCartesianOffsetUnits=m  TranslationROffset=0  TranslationROffsetUnits=m  TranslationZOffset=0  TranslationZOffsetUnits=m  TranslationThetaOffset=0  TranslationThetaOffsetUnits=deg  RotationMethod=None  RotationAngleUnits=deg  RotationStandardAxis=+Z  RotationAngle=0.0  RotationArbitraryAxis=[0 0 1]  FollAlignAxisA=+X  BaseAlignAxisA=+Y  FollAlignAxisB=+Y  BaseAlignAxisB=+Z  RotationSequenceAxes=FollowerAxes  RotationSequence=XYX  RotationSequenceAngles=[0 0 0]  RotationSequenceAnglesUnits=deg  RotationMatrix=[1 0 0; 0 1 0; 0 0 1]  Quaternion=[1 0 0 0]
  Rigid Transform2 : sm_lib/Frames and Transforms/Rigid Transform  TranslationMethod=None  TranslationStandardOffset=0  TranslationStandardOffsetUnits=m  TranslationStandardAxis=+Z  TranslationCartesianOffset=[0 0 0]  TranslationCartesianOffsetUnits=m  TranslationROffset=0  TranslationROffsetUnits=m  TranslationZOffset=0  TranslationZOffsetUnits=m  TranslationThetaOffset=0  TranslationThetaOffsetUnits=deg  RotationMethod=None  RotationAngleUnits=deg  RotationStandardAxis=+Z  RotationAngle=0.0  RotationArbitraryAxis=[0 0 1]  FollAlignAxisA=+X  BaseAlignAxisA=+Y  FollAlignAxisB=+Y  BaseAlignAxisB=+Z  RotationSequenceAxes=FollowerAxes  RotationSequence=XYX  RotationSequenceAngles=[0 0 0]  RotationSequenceAnglesUnits=deg  RotationMatrix=[1 0 0; 0 1 0; 0 0 1]  Quaternion=[1 0 0 0]
  Spatial Contact Force : sm_lib/Forces and Torques/Spatial Contact Force  SenseContactBaseRotation=off  SenseContactBaseTranslation=off  CoefficientOfDynamicFriction=mu_k  CoefficientOfStaticFriction=mu_s  NormalDamping=contact_damping  NormalDampingUnits=N/(m/s)  SenseContactSignal=off  NormalStiffness=contact_stiffness  NormalStiffnessUnits=N/m  FrictionalCriticalVelocity=mu_vth  FrictionalCriticalVelocityUnits=m/s  ZeroCrossDetectContactStartAndEnd=off  SenseContactFollowerRotation=off  SenseContactFollowerTranslation=off  FrictionType=SmoothStickSlip  SenseFrictionalForceMagnitude=on  SenseNormalForceMagnitude=on  NormalForceType=SmoothSpringDamper  SenseNormalVelocity=off  SensePenetrationDepth=off  SenseSeparationDistance=off  SenseTangentialVelocity=off  NormalTransitionRegionWidth=1e-4  NormalTransitionRegionWidthUnits=m
  Spatial Contact Force1 : sm_lib/Forces and Torques/Spatial Contact Force  SenseContactBaseRotation=off  SenseContactBaseTranslation=off  CoefficientOfDynamicFriction=mu_k  CoefficientOfStaticFriction=mu_s  NormalDamping=contact_damping  NormalDampingUnits=N/(m/s)  SenseContactSignal=off  NormalStiffness=contact_stiffness  NormalStiffnessUnits=N/m  FrictionalCriticalVelocity=mu_vth  FrictionalCriticalVelocityUnits=m/s  ZeroCrossDetectContactStartAndEnd=off  SenseContactFollowerRotation=off  SenseContactFollowerTranslation=off  FrictionType=SmoothStickSlip  SenseFrictionalForceMagnitude=on  SenseNormalForceMagnitude=on  NormalForceType=SmoothSpringDamper  SenseNormalVelocity=off  SensePenetrationDepth=off  SenseSeparationDistance=off  SenseTangentialVelocity=off  NormalTransitionRegionWidth=1e-4  NormalTransitionRegionWidthUnits=m
  Spatial Contact Force2 : sm_lib/Forces and Torques/Spatial Contact Force  SenseContactBaseRotation=off  SenseContactBaseTranslation=off  CoefficientOfDynamicFriction=mu_k  CoefficientOfStaticFriction=mu_s  NormalDamping=contact_damping  NormalDampingUnits=N/(m/s)  SenseContactSignal=off  NormalStiffness=contact_stiffness  NormalStiffnessUnits=N/m  FrictionalCriticalVelocity=mu_vth  FrictionalCriticalVelocityUnits=m/s  ZeroCrossDetectContactStartAndEnd=off  SenseContactFollowerRotation=off  SenseContactFollowerTranslation=off  FrictionType=SmoothStickSlip  SenseFrictionalForceMagnitude=on  SenseNormalForceMagnitude=on  NormalForceType=SmoothSpringDamper  SenseNormalVelocity=off  SensePenetrationDepth=off  SenseSeparationDistance=off  SenseTangentialVelocity=off  NormalTransitionRegionWidth=1e-4  NormalTransitionRegionWidthUnits=m
  Spherical Solid : sm_lib/Body Elements/Spherical Solid  GraphicAmbientColor=[0.15 0.15 0.15 1.0]  BasedOnType=Mass  CenterOfMass=[0 0 0]  CenterOfMassUnits=m  GraphicDiffuseColor=[0.5 0.5 0.5]  Density=1000  DensityUnits=kg/m^3  DoExposeReferenceFrame=on  GraphicEmissiveColor=[0.0 0.0 0.0 1.0]  ExportEntireGeometry=on  SerializedExposedGeometries=<exposedGeometries><exposedGeom><rawGeomId>entire</rawGeomId><exposedGeomId>G</exposedGeomId></exposedGeom></exposedGeometries>  SerializedFrames=<Frames/>  MarkerShape=Sphere  MarkerSize=10  GraphicType=FromGeometry  InertiaType=CalculateFromGeometry  Mass=0  MassUnits=g  MomentsOfInertia=[1 1 1]  MomentsOfInertiaUnits=kg*m^2  GraphicOpacity=1.0  ProductsOfInertia=[0 0 0]  ProductsOfInertiaUnits=kg*m^2  GraphicShininess=75  GraphicSpecularColor=[0.5 0.5 0.5 1.0]  SphereRadius=foot_z/2  SphereRadiusUnits=cm  GraphicVisPropType=SimpleVisualProperties
  Spherical Solid1 : sm_lib/Body Elements/Spherical Solid  GraphicAmbientColor=[0.15 0.15 0.15 1.0]  BasedOnType=Mass  CenterOfMass=[0 0 0]  CenterOfMassUnits=m  GraphicDiffuseColor=[0.5 0.5 0.5]  Density=1000  DensityUnits=kg/m^3  DoExposeReferenceFrame=on  GraphicEmissiveColor=[0.0 0.0 0.0 1.0]  ExportEntireGeometry=on  SerializedExposedGeometries=<exposedGeometries><exposedGeom><rawGeomId>entire</rawGeomId><exposedGeomId>G</exposedGeomId></exposedGeom></exposedGeometries>  SerializedFrames=<Frames/>  MarkerShape=Sphere  MarkerSize=10  GraphicType=FromGeometry  InertiaType=CalculateFromGeometry  Mass=0  MassUnits=g  MomentsOfInertia=[1 1 1]  MomentsOfInertiaUnits=kg*m^2  GraphicOpacity=1.0  ProductsOfInertia=[0 0 0]  ProductsOfInertiaUnits=kg*m^2  GraphicShininess=75  GraphicSpecularColor=[0.5 0.5 0.5 1.0]  SphereRadius=foot_z/2  SphereRadiusUnits=cm  GraphicVisPropType=SimpleVisualProperties
  Spherical Solid2 : sm_lib/Body Elements/Spherical Solid  GraphicAmbientColor=[0.15 0.15 0.15 1.0]  BasedOnType=Mass  CenterOfMass=[0 0 0]  CenterOfMassUnits=m  GraphicDiffuseColor=[0.5 0.5 0.5]  Density=1000  DensityUnits=kg/m^3  DoExposeReferenceFrame=on  GraphicEmissiveColor=[0.0 0.0 0.0 1.0]  ExportEntireGeometry=on  SerializedExposedGeometries=<exposedGeometries><exposedGeom><rawGeomId>entire</rawGeomId><exposedGeomId>G</exposedGeomId></exposedGeom></exposedGeometries>  SerializedFrames=<Frames/>  MarkerShape=Sphere  MarkerSize=10  GraphicType=FromGeometry  InertiaType=CalculateFromGeometry  Mass=0  MassUnits=g  MomentsOfInertia=[1 1 1]  MomentsOfInertiaUnits=kg*m^2  GraphicOpacity=1.0  ProductsOfInertia=[0 0 0]  ProductsOfInertiaUnits=kg*m^2  GraphicShininess=75  GraphicSpecularColor=[0.5 0.5 0.5 1.0]  SphereRadius=foot_z/2  SphereRadiusUnits=cm  GraphicVisPropType=SimpleVisualProperties
  Upper Leg to Hip : sm_lib/Frames and Transforms/Rigid Transform  TranslationMethod=Cartesian  TranslationStandardOffset=0  TranslationStandardOffsetUnits=cm  TranslationStandardAxis=+Z  TranslationCartesianOffset=[0 0 upper_leg_length/2]  TranslationCartesianOffsetUnits=cm  TranslationROffset=0  TranslationROffsetUnits=m  TranslationZOffset=0  TranslationZOffsetUnits=m  TranslationThetaOffset=0  TranslationThetaOffsetUnits=deg  RotationMethod=StandardAxis  RotationAngleUnits=deg  RotationStandardAxis=+X  RotationAngle=90  RotationArbitraryAxis=[0 0 1]  FollAlignAxisA=+X  BaseAlignAxisA=+Y  FollAlignAxisB=+Y  BaseAlignAxisB=+Z  RotationSequenceAxes=FollowerAxes  RotationSequence=XYX  RotationSequenceAngles=[0 0 0]  RotationSequenceAnglesUnits=deg  RotationMatrix=[1 0 0; 0 1 0; 0 0 1]  Quaternion=[1 0 0 0]
  Upper Leg to Hip1 : sm_lib/Frames and Transforms/Rigid Transform  TranslationMethod=Cartesian  TranslationStandardOffset=0  TranslationStandardOffsetUnits=cm  TranslationStandardAxis=+Z  TranslationCartesianOffset=[0 0 upper_leg_length/2]  TranslationCartesianOffsetUnits=cm  TranslationROffset=0  TranslationROffsetUnits=m  TranslationZOffset=0  TranslationZOffsetUnits=m  TranslationThetaOffset=0  TranslationThetaOffsetUnits=deg  RotationMethod=StandardAxis  RotationAngleUnits=deg  RotationStandardAxis=+X  RotationAngle=90  RotationArbitraryAxis=[0 0 1]  FollAlignAxisA=+X  BaseAlignAxisA=+Y  FollAlignAxisB=+Y  BaseAlignAxisB=+Z  RotationSequenceAxes=FollowerAxes  RotationSequence=XYX  RotationSequenceAngles=[0 0 0]  RotationSequenceAnglesUnits=deg  RotationMatrix=[1 0 0; 0 1 0; 0 0 1]  Quaternion=[1 0 0 0]
  Upper Leg1 : sm_lib/Body Elements/Cylindrical Solid  GraphicAmbientColor=[0.15 0.15 0.15 1.0]  BasedOnType=Density  CenterOfMass=[0 0 0]  CenterOfMassUnits=m  GraphicDiffuseColor=[1.0 0.4 0.4]  CylinderLength=upper_leg_length  CylinderLengthUnits=cm  CylinderRadius=leg_radius  CylinderRadiusUnits=cm  Density=density  DensityUnits=kg/m^3  DoExposeReferenceFrame=on  GraphicEmissiveColor=[0.0 0.0 0.0 1.0]  ExportEntireGeometry=off  SerializedFrames=<Frames/>  MarkerShape=Sphere  MarkerSize=10  GraphicType=FromGeometry  InertiaType=CalculateFromGeometry  Mass=1  MassUnits=kg  MomentsOfInertia=[1 1 1]  MomentsOfInertiaUnits=kg*m^2  GraphicOpacity=1.0  ProductsOfInertia=[1 1 1]  ProductsOfInertiaUnits=kg*m^2  GraphicShininess=75  GraphicSpecularColor=[0.5 0.5 0.5 1.0]  GraphicVisPropType=SimpleVisualProperties
  H : PMIOPort  Side=Right
  G : PMIOPort  Port=2  Side=Right
  meas : Outport  VectorParamsAs1DForOutWhenUnconnected=off
  wires:
  Demux/3 -> Hip Joint/1
  Demux/2 -> Knee Joint/1
  Demux/1 -> Ankle Joint/1
  Ankle Joint/1 -> Package Measurements/3(ankle)
  Knee Joint/1 -> Package Measurements/4(knee)
  Hip Joint/1 -> Package Measurements/5(hip)
  torques/1 -> Demux/1
  Package Measurements/1(meas) -> meas/1
  Knee Joint1/1 -> Package Measurements/6(seg4)
  Demux/4 -> Knee Joint1/1
  Foot and Contact/1(Fn) -> Add/1
  PS-Simulink Converter/1 -> Add/2
  PS-Simulink Converter1/1 -> Add/3
  Add/1 -> Package Measurements/1(Fn)
  Foot and Contact/2(Ff) -> Add1/1
  PS-Simulink Converter2/1 -> Add1/2
  PS-Simulink Converter3/1 -> Add1/3
  Add1/1 -> Package Measurements/2(Ff)
  PS-Simulink Converter4/1 -> Add/4
  PS-Simulink Converter5/1 -> Add1/4
  connections:
  G/RConn1 -- Spatial Contact Force/LConn1 -- Spatial Contact Force2/LConn1 -- Spatial Contact Force1/LConn1 -- Foot and Contact/LConn1
  Foot and Contact/RConn1 -- Foot Offset/LConn1
  Ankle Joint/LConn1 -- Foot Offset/RConn1
  Hip Joint/RConn1 -- Hip to World Coords/LConn1
  Ankle Joint/RConn1 -- Ankle to Lower Leg/LConn1
  Knee to Upper Leg/LConn1 -- Knee Joint/RConn1
  Lower Leg/RConn1 -- Ankle to Lower Leg/RConn1 -- Lower Leg to Knee/LConn1
  Upper Leg to Hip/LConn1 -- Knee to Upper Leg/RConn1 -- Lower Leg1/RConn1
  Knee Joint/LConn1 -- Lower Leg to Knee/RConn1
  Hip to World Coords/RConn1 -- H/RConn1
  Spatial Contact Force/RConn1 -- Spherical Solid/LConn1
  Upper Leg to Hip1/LConn1 -- Lower Leg2/RConn1 -- Knee to Upper Leg1/RConn1
  Upper Leg to Hip/RConn1 -- Knee Joint1/LConn1
  Knee to Upper Leg1/LConn1 -- Knee Joint1/RConn1
  Upper Leg to Hip1/RConn1 -- Hip Joint/LConn1
  Spatial Contact Force1/RConn1 -- Spherical Solid1/LConn1
  Spherical Solid/RConn1 -- Rigid Transform/LConn1
  Lower Leg/LConn1 -- Rigid Transform/RConn1
  Spherical Solid1/RConn1 -- Rigid Transform1/LConn1
  Rigid Transform1/RConn1 -- Lower Leg1/LConn1
  Spatial Contact Force/RConn2 -- PS-Simulink Converter/LConn1
  PS-Simulink Converter1/LConn1 -- Spatial Contact Force1/RConn2
  Spatial Contact Force/RConn3 -- PS-Simulink Converter2/LConn1
  Spatial Contact Force1/RConn3 -- PS-Simulink Converter3/LConn1
  Rigid Transform2/LConn1 -- Spherical Solid2/RConn1
  Rigid Transform2/RConn1 -- Lower Leg2/LConn1
  Spatial Contact Force2/RConn1 -- Spherical Solid2/LConn1
  Spatial Contact Force2/RConn2 -- PS-Simulink Converter4/LConn1
  Spatial Contact Force2/RConn3 -- PS-Simulink Converter5/LConn1

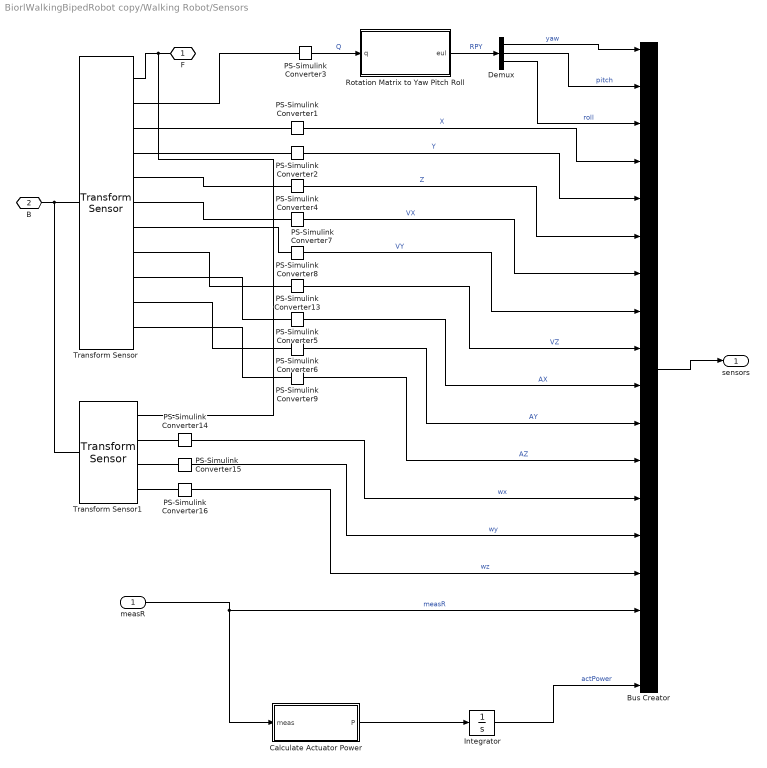
== system BiorlWalkingBipedRobot copy/Walking Robot/Sensors ==
  measR : Inport
  Bus Creator : BusCreator  Inputs=18
  Calculate Actuator Power : Subsystem
  Demux : Demux  Outputs=3
  Integrator : Integrator
  PS-Simulink Converter{1..9,13..16} (13 alike) : nesl_utility/PS-Simulink Converter  PhysicalDomain=network_engine_domain  SubClassName=ps_output  LeftPortType=input  RightPortType=output  PseudoPeriodic=off  Frequencies=[]  VectorFormat=1-D array  Unit=1  AffineConversion=off
  Rotation Matrix to Yaw Pitch Roll : MATLAB Function  TreatAsAtomicUnit=on
  Transform Sensor : sm_lib/Frames and Transforms/Transform Sensor  MeasurementFrame=World  RotationSequence=XYX  SenseAngle=off  SenseAxis=off  SenseQ=on  SenseR=off  SenseRotationSequence=off  SenseOmegaX=off  SenseOmegaY=off  SenseOmegaZ=off  SenseOmega=off  SenseQDot=off  SenseRDot=off  SenseRotationSequenceDot=off  SenseAlphaX=off  SenseAlphaY=off  SenseAlphaZ=off  SenseAlpha=off  SenseQDDot=off  SenseRDDot=off  SenseX=on  SenseY=on  SenseZ=on  SenseXYZ=off  SenseRad=off  SenseAzim=off  SenseDist=off  SenseInc=off  SenseXDot=on  SenseYDot=on  SenseZDot=on  SenseXYZDot=off  SenseRadDot=off  SenseAzimDot=off  SenseDistDot=off  SenseIncDot=off  SenseXDDot=on  SenseYDDot=on  SenseZDDot=on  SenseXYZDDot=off  SenseRadDDot=off  SenseAzimDDot=off  SenseDistDDot=off  SenseIncDDot=off
  Transform Sensor1 : sm_lib/Frames and Transforms/Transform Sensor  MeasurementFrame=NonRotatingFollower  RotationSequence=XYX  SenseAngle=off  SenseAxis=off  SenseQ=off  SenseR=off  SenseRotationSequence=off  SenseOmegaX=on  SenseOmegaY=on  SenseOmegaZ=on  SenseOmega=off  SenseQDot=off  SenseRDot=off  SenseRotationSequenceDot=off  SenseAlphaX=off  SenseAlphaY=off  SenseAlphaZ=off  SenseAlpha=off  SenseQDDot=off  SenseRDDot=off  SenseX=off  SenseY=off  SenseZ=off  SenseXYZ=off  SenseRad=off  SenseAzim=off  SenseDist=off  SenseInc=off  SenseXDot=off  SenseYDot=off  SenseZDot=off  SenseXYZDot=off  SenseRadDot=off  SenseAzimDot=off  SenseDistDot=off  SenseIncDot=off  SenseXDDot=off  SenseYDDot=off  SenseZDDot=off  SenseXYZDDot=off  SenseRadDDot=off  SenseAzimDDot=off  SenseDistDDot=off  SenseIncDDot=off
  F : PMIOPort  Side=Right
  B : PMIOPort  Port=2  Side=Left
  sensors : Outport  VectorParamsAs1DForOutWhenUnconnected=off
  wires:
  PS-Simulink Converter2/1 -> Bus Creator/5  "Y"
  PS-Simulink Converter4/1 -> Bus Creator/6  "Z"
  PS-Simulink Converter5/1 -> Bus Creator/10  "AX"
  Bus Creator/1 -> sensors/1
  PS-Simulink Converter3/1 -> Rotation Matrix to Yaw Pitch Roll/1(q)  "Q"
  PS-Simulink Converter1/1 -> Bus Creator/4  "X"
  PS-Simulink Converter6/1 -> Bus Creator/11  "AY"
  PS-Simulink Converter7/1 -> Bus Creator/7  "VX"
  PS-Simulink Converter8/1 -> Bus Creator/8  "VY"
  PS-Simulink Converter9/1 -> Bus Creator/12  "AZ"
  PS-Simulink Converter13/1 -> Bus Creator/9  "VZ"
  Rotation Matrix to Yaw Pitch Roll/1(eul) -> Demux/1  "RPY"
  Demux/3 -> Bus Creator/3  "roll"
  Demux/2 -> Bus Creator/2  "pitch"
  Demux/1 -> Bus Creator/1  "yaw"
  PS-Simulink Converter14/1 -> Bus Creator/13  "wx"
  PS-Simulink Converter15/1 -> Bus Creator/14  "wy"
  PS-Simulink Converter16/1 -> Bus Creator/15  "wz"
  measR/1 -> Calculate Actuator Power/1(meas), Bus Creator/16  "measR"
  Integrator/1 -> Bus Creator/18  "actPower"
  Calculate Actuator Power/1(P) -> Integrator/1
  connections:
  PS-Simulink Converter1/LConn1 -- Transform Sensor/RConn3
  PS-Simulink Converter3/LConn1 -- Transform Sensor/RConn2
  Transform Sensor/RConn1 -- Transform Sensor1/RConn1 -- F/RConn1
  Transform Sensor/RConn5 -- PS-Simulink Converter4/LConn1
  Transform Sensor/RConn4 -- PS-Simulink Converter2/LConn1
  Transform Sensor/LConn1 -- Transform Sensor1/LConn1 -- B/RConn1
  PS-Simulink Converter7/LConn1 -- Transform Sensor/RConn6
  PS-Simulink Converter14/LConn1 -- Transform Sensor1/RConn2
  PS-Simulink Converter15/LConn1 -- Transform Sensor1/RConn3
  Transform Sensor1/RConn4 -- PS-Simulink Converter16/LConn1
  Transform Sensor/RConn7 -- PS-Simulink Converter8/LConn1
  PS-Simulink Converter13/LConn1 -- Transform Sensor/RConn8
  PS-Simulink Converter5/LConn1 -- Transform Sensor/RConn9
  Transform Sensor/RConn10 -- PS-Simulink Converter6/LConn1
  PS-Simulink Converter9/LConn1 -- Transform Sensor/RConn11
